simulink model "case2"  (R2024b)
settings: Solver=FixedStepAuto  StartTime=0  StopTime=1  FixedStep=1e-7  RelTol=1e-3
values from neighbouring files (symbols this model uses):
  SG_D_1_D = 0.01056    [IEEE9_case_parameters.m]    (also in case1_parameters.m; case2_parameters.m; case3_parameters.m; case4_parameters.m)
  SG_D_1_EnableSaturation = 0    [IEEE9_case_parameters.m]    (also in case1_parameters.m; case2_parameters.m; case3_parameters.m; case4_parameters.m)
  SG_D_1_f0 = 60    [IEEE9_case_parameters.m]    (also in case1_parameters.m; case2_parameters.m; case3_parameters.m; case4_parameters.m)
  SG_D_1_H = 7.5    [IEEE9_case_parameters.m]    (also in case1_parameters.m; case2_parameters.m; case3_parameters.m; case4_parameters.m)
  SG_D_1_K_A = 20    [IEEE9_case_parameters.m]    (also in case1_parameters.m; case2_parameters.m; case3_parameters.m; case4_parameters.m)
  SG_D_1_K_E = 1.000000e+1    (= 10)    [IEEE9_case_parameters.m]    (also in case1_parameters.m; case2_parameters.m; case3_parameters.m; case4_parameters.m)
  SG_D_1_K_F = 2.363    [IEEE9_case_parameters.m]    (also in case1_parameters.m; case2_parameters.m; case3_parameters.m; case4_parameters.m)
  SG_D_1_K_s = 0.5    [IEEE9_case_parameters.m]    (also in case1_parameters.m = 5; case2_parameters.m = 5; case3_parameters.m = 5; case4_parameters.m = 5)
  SG_D_1_R_a = 0.001088    [IEEE9_case_parameters.m]    (also in case1_parameters.m; case2_parameters.m; case3_parameters.m; case4_parameters.m)
  SG_D_1_S_A = 1    [IEEE9_case_parameters.m]    (also in case1_parameters.m; case2_parameters.m; case3_parameters.m; case4_parameters.m)
  SG_D_1_S_B = 0.103    [IEEE9_case_parameters.m]    (also in case1_parameters.m; case2_parameters.m; case3_parameters.m; case4_parameters.m)
  SG_D_1_S_N = 10.659857    [IEEE9_case_parameters.m]    (also in case1_parameters.m; case2_parameters.m; case3_parameters.m; case4_parameters.m)
  SG_D_1_SpeedPara = 200    [IEEE9_case_parameters.m]    (also in case1_parameters.m; case2_parameters.m; case3_parameters.m; case4_parameters.m)
  SG_D_1_T_0 = 0.720173    [IEEE9_case_parameters.m]    (also in case1_parameters.m = 0.755522; case2_parameters.m = 0.808931; case3_parameters.m = 0.869402; case4_parameters.m = 0.729316)
  SG_D_1_T_1 = 0.3    [IEEE9_case_parameters.m]    (also in case1_parameters.m; case2_parameters.m; case3_parameters.m; case4_parameters.m)
  SG_D_1_T_2 = 0.05    [IEEE9_case_parameters.m]    (also in case1_parameters.m; case2_parameters.m; case3_parameters.m; case4_parameters.m)
  SG_D_1_T_3 = 0.02    [IEEE9_case_parameters.m]    (also in case1_parameters.m; case2_parameters.m; case3_parameters.m; case4_parameters.m)
  SG_D_1_T_4 = 0.005    [IEEE9_case_parameters.m]    (also in case1_parameters.m; case2_parameters.m; case3_parameters.m; case4_parameters.m)
  SG_D_1_T_A = 0.02    [IEEE9_case_parameters.m]    (also in case1_parameters.m; case2_parameters.m; case3_parameters.m; case4_parameters.m)
  SG_D_1_T_dd = 8.000000e+0    (= 8)    [IEEE9_case_parameters.m]    (also in case1_parameters.m; case2_parameters.m; case3_parameters.m; case4_parameters.m)
  SG_D_1_T_ddd = 0.04    [IEEE9_case_parameters.m]    (also in case1_parameters.m; case2_parameters.m; case3_parameters.m; case4_parameters.m)
  SG_D_1_T_E = 0.314    [IEEE9_case_parameters.m]    (also in case1_parameters.m; case2_parameters.m; case3_parameters.m; case4_parameters.m)
  SG_D_1_T_F = 0.35    [IEEE9_case_parameters.m]    (also in case1_parameters.m; case2_parameters.m; case3_parameters.m; case4_parameters.m)
  SG_D_1_T_qd = 0.8    [IEEE9_case_parameters.m]    (also in case1_parameters.m; case2_parameters.m; case3_parameters.m; case4_parameters.m)
  SG_D_1_T_qdd = 0.02    [IEEE9_case_parameters.m]    (also in case1_parameters.m; case2_parameters.m; case3_parameters.m; case4_parameters.m)
  SG_D_1_T_speed = 0.1    [IEEE9_case_parameters.m]    (also in case1_parameters.m = 200; case2_parameters.m = 200; case3_parameters.m = 200; case4_parameters.m = 200)
  SG_D_1_T_w = 0.5    [IEEE9_case_parameters.m]    (also in case1_parameters.m; case2_parameters.m; case3_parameters.m; case4_parameters.m)
  SG_D_1_V_ref = 1.990276    [IEEE9_case_parameters.m]    (also in case1_parameters.m = 2.042296; case2_parameters.m = 2.051388; case3_parameters.m = 2.089584; case4_parameters.m = 2.01845)
  SG_D_1_w_ref = 376.991118    [IEEE9_case_parameters.m]    (also in case1_parameters.m; case2_parameters.m; case3_parameters.m; case4_parameters.m)
  SG_D_1_wb = 6.000000e+1    (= 60)    [IEEE9_case_parameters.m]    (also in case1_parameters.m; case2_parameters.m; case3_parameters.m; case4_parameters.m)
  SG_D_1_x_d = 1.9    [IEEE9_case_parameters.m]    (also in case1_parameters.m; case2_parameters.m; case3_parameters.m; case4_parameters.m)
  SG_D_1_x_dd = 0.302    [IEEE9_case_parameters.m]    (also in case1_parameters.m; case2_parameters.m; case3_parameters.m; case4_parameters.m)
  SG_D_1_x_ddd = 0.204    [IEEE9_case_parameters.m]    (also in case1_parameters.m; case2_parameters.m; case3_parameters.m; case4_parameters.m)
  SG_D_1_x_l = 0.05    [IEEE9_case_parameters.m]    (also in case1_parameters.m; case2_parameters.m; case3_parameters.m; case4_parameters.m)
  SG_D_1_x_q = 1.3    [IEEE9_case_parameters.m]    (also in case1_parameters.m; case2_parameters.m; case3_parameters.m; case4_parameters.m)
  SG_D_1_x_qd = 0.5    [IEEE9_case_parameters.m]    (also in case1_parameters.m; case2_parameters.m; case3_parameters.m; case4_parameters.m)
  SG_D_1_x_qdd = 0.3    [IEEE9_case_parameters.m]    (also in case1_parameters.m; case2_parameters.m; case3_parameters.m; case4_parameters.m)
  SG_D_2_D = 0.02    [IEEE9_case_parameters.m]    (also in case1_parameters.m; case2_parameters.m; case3_parameters.m; case4_parameters.m)
  SG_D_2_EnableSaturation = 0    [IEEE9_case_parameters.m]    (also in case1_parameters.m; case2_parameters.m; case3_parameters.m; case4_parameters.m)
  SG_D_2_f0 = 60    [IEEE9_case_parameters.m]    (also in case1_parameters.m; case2_parameters.m; case3_parameters.m; case4_parameters.m)
  SG_D_2_H = 8.000000e+0    (= 8)    [IEEE9_case_parameters.m]    (also in case1_parameters.m; case2_parameters.m; case3_parameters.m; case4_parameters.m)
  SG_D_2_K_A = 20    [IEEE9_case_parameters.m]    (also in case1_parameters.m; case2_parameters.m; case3_parameters.m; case4_parameters.m)
  SG_D_2_K_E = 1.000000e+1    (= 10)    [IEEE9_case_parameters.m]    (also in case1_parameters.m; case2_parameters.m; case3_parameters.m; case4_parameters.m)
  SG_D_2_K_F = 2.363    [IEEE9_case_parameters.m]    (also in case1_parameters.m; case2_parameters.m; case3_parameters.m; case4_parameters.m)
  SG_D_2_K_s = 0.5    [IEEE9_case_parameters.m]    (also in case1_parameters.m = 4; case2_parameters.m = 4; case3_parameters.m = 4; case4_parameters.m = 4)
  SG_D_2_R_a = 0.001088    [IEEE9_case_parameters.m]    (also in case1_parameters.m; case2_parameters.m; case3_parameters.m; case4_parameters.m)
  SG_D_2_S_A = 1    [IEEE9_case_parameters.m]    (also in case1_parameters.m; case2_parameters.m; case3_parameters.m; case4_parameters.m)
  SG_D_2_S_B = 0.103    [IEEE9_case_parameters.m]    (also in case1_parameters.m; case2_parameters.m; case3_parameters.m; case4_parameters.m)
  SG_D_2_S_N = 10.659857    [IEEE9_case_parameters.m]    (also in case1_parameters.m; case2_parameters.m; case3_parameters.m; case4_parameters.m)
  SG_D_2_SpeedPara = 200    [IEEE9_case_parameters.m]    (also in case1_parameters.m; case2_parameters.m; case3_parameters.m; case4_parameters.m)
  SG_D_2_T_0 = 1.632913    [IEEE9_case_parameters.m]    (also in case1_parameters.m = 1.632925; case2_parameters.m = 1.632915; case3_parameters.m = 1.632914; case4_parameters.m = 1.632927)
  SG_D_2_T_1 = 0.2    [IEEE9_case_parameters.m]    (also in case1_parameters.m; case2_parameters.m; case3_parameters.m; case4_parameters.m)
  SG_D_2_T_2 = 0.05    [IEEE9_case_parameters.m]    (also in case1_parameters.m; case2_parameters.m; case3_parameters.m; case4_parameters.m)
  SG_D_2_T_3 = 0.02    [IEEE9_case_parameters.m]    (also in case1_parameters.m; case2_parameters.m; case3_parameters.m; case4_parameters.m)
  SG_D_2_T_4 = 0.005    [IEEE9_case_parameters.m]    (also in case1_parameters.m; case2_parameters.m; case3_parameters.m; case4_parameters.m)
  SG_D_2_T_A = 0.02    [IEEE9_case_parameters.m]    (also in case1_parameters.m; case2_parameters.m; case3_parameters.m; case4_parameters.m)
  SG_D_2_T_dd = 7.9    [IEEE9_case_parameters.m]    (also in case1_parameters.m; case2_parameters.m; case3_parameters.m; case4_parameters.m)
  SG_D_2_T_ddd = 0.04    [IEEE9_case_parameters.m]    (also in case1_parameters.m; case2_parameters.m; case3_parameters.m; case4_parameters.m)
  SG_D_2_T_E = 0.314    [IEEE9_case_parameters.m]    (also in case1_parameters.m; case2_parameters.m; case3_parameters.m; case4_parameters.m)
  SG_D_2_T_F = 0.35    [IEEE9_case_parameters.m]    (also in case1_parameters.m; case2_parameters.m; case3_parameters.m; case4_parameters.m)
  SG_D_2_T_qd = 0.8    [IEEE9_case_parameters.m]    (also in case1_parameters.m; case2_parameters.m; case3_parameters.m; case4_parameters.m)
  SG_D_2_T_qdd = 0.015    [IEEE9_case_parameters.m]    (also in case1_parameters.m; case2_parameters.m; case3_parameters.m; case4_parameters.m)
  SG_D_2_T_speed = 0.1    [IEEE9_case_parameters.m]    (also in case1_parameters.m = 150; case2_parameters.m = 150; case3_parameters.m = 150; case4_parameters.m = 150)
  SG_D_2_T_w = 0.35    [IEEE9_case_parameters.m]    (also in case1_parameters.m; case2_parameters.m; case3_parameters.m; case4_parameters.m)
  SG_D_2_V_ref = 2.58547    [IEEE9_case_parameters.m]    (also in case1_parameters.m = 2.597896; case2_parameters.m = 2.587136; case3_parameters.m = 2.586042; case4_parameters.m = 2.599679)
  SG_D_2_w_ref = 376.991118    [IEEE9_case_parameters.m]    (also in case1_parameters.m; case2_parameters.m; case3_parameters.m; case4_parameters.m)
  SG_D_2_wb = 6.000000e+1    (= 60)    [IEEE9_case_parameters.m]    (also in case1_parameters.m; case2_parameters.m; case3_parameters.m; case4_parameters.m)
  SG_D_2_x_d = 1.8    [IEEE9_case_parameters.m]    (also in case1_parameters.m; case2_parameters.m; case3_parameters.m; case4_parameters.m)
  SG_D_2_x_dd = 0.302    [IEEE9_case_parameters.m]    (also in case1_parameters.m; case2_parameters.m; case3_parameters.m; case4_parameters.m)
  SG_D_2_x_ddd = 0.204    [IEEE9_case_parameters.m]    (also in case1_parameters.m; case2_parameters.m; case3_parameters.m; case4_parameters.m)
  SG_D_2_x_l = 0.05    [IEEE9_case_parameters.m]    (also in case1_parameters.m; case2_parameters.m; case3_parameters.m; case4_parameters.m)
  SG_D_2_x_q = 1.25    [IEEE9_case_parameters.m]    (also in case1_parameters.m; case2_parameters.m; case3_parameters.m; case4_parameters.m)
  SG_D_2_x_qd = 0.5    [IEEE9_case_parameters.m]    (also in case1_parameters.m; case2_parameters.m; case3_parameters.m; case4_parameters.m)
  SG_D_2_x_qdd = 0.3    [IEEE9_case_parameters.m]    (also in case1_parameters.m; case2_parameters.m; case3_parameters.m; case4_parameters.m)
  SG_D_3_D = 0.02    [IEEE9_case_parameters.m]    (also in case1_parameters.m; case2_parameters.m; case3_parameters.m; case4_parameters.m)
  SG_D_3_EnableSaturation = 0    [IEEE9_case_parameters.m]    (also in case1_parameters.m; case2_parameters.m; case3_parameters.m; case4_parameters.m)
  SG_D_3_f0 = 60    [IEEE9_case_parameters.m]    (also in case1_parameters.m; case2_parameters.m; case3_parameters.m; case4_parameters.m)
  SG_D_3_H = 7.7    [IEEE9_case_parameters.m]    (also in case1_parameters.m; case2_parameters.m; case3_parameters.m; case4_parameters.m)
  SG_D_3_K_A = 20    [IEEE9_case_parameters.m]    (also in case1_parameters.m; case2_parameters.m; case3_parameters.m; case4_parameters.m)
  SG_D_3_K_E = 1.000000e+1    (= 10)    [IEEE9_case_parameters.m]    (also in case1_parameters.m; case2_parameters.m; case3_parameters.m; case4_parameters.m)
  SG_D_3_K_F = 2.363    [IEEE9_case_parameters.m]    (also in case1_parameters.m; case2_parameters.m; case3_parameters.m; case4_parameters.m)
  SG_D_3_K_s = 0.2    [IEEE9_case_parameters.m]    (also in case1_parameters.m = 2; case2_parameters.m = 2; case3_parameters.m = 2; case4_parameters.m = 2)
  SG_D_3_R_a = 0.001088    [IEEE9_case_parameters.m]    (also in case1_parameters.m; case2_parameters.m; case3_parameters.m; case4_parameters.m)
  SG_D_3_S_A = 1    [IEEE9_case_parameters.m]    (also in case1_parameters.m; case2_parameters.m; case3_parameters.m; case4_parameters.m)
  SG_D_3_S_B = 0.103    [IEEE9_case_parameters.m]    (also in case1_parameters.m; case2_parameters.m; case3_parameters.m; case4_parameters.m)
  SG_D_3_S_N = 10.659857    [IEEE9_case_parameters.m]    (also in case1_parameters.m; case2_parameters.m; case3_parameters.m; case4_parameters.m)
  SG_D_3_SpeedPara = 200    [IEEE9_case_parameters.m]    (also in case1_parameters.m; case2_parameters.m; case3_parameters.m; case4_parameters.m)
  SG_D_3_T_0 = 0.850788    [IEEE9_case_parameters.m]    (also in case1_parameters.m = 0.850786; case2_parameters.m = 0.850787; case3_parameters.m; case4_parameters.m = 0.850786)
  SG_D_3_T_1 = 0.2    [IEEE9_case_parameters.m]    (also in case1_parameters.m; case2_parameters.m; case3_parameters.m; case4_parameters.m)
  SG_D_3_T_2 = 0.05    [IEEE9_case_parameters.m]    (also in case1_parameters.m; case2_parameters.m; case3_parameters.m; case4_parameters.m)
  SG_D_3_T_3 = 0.02    [IEEE9_case_parameters.m]    (also in case1_parameters.m; case2_parameters.m; case3_parameters.m; case4_parameters.m)
  SG_D_3_T_4 = 0.005    [IEEE9_case_parameters.m]    (also in case1_parameters.m; case2_parameters.m; case3_parameters.m; case4_parameters.m)
  SG_D_3_T_A = 0.02    [IEEE9_case_parameters.m]    (also in case1_parameters.m; case2_parameters.m; case3_parameters.m; case4_parameters.m)
  SG_D_3_T_dd = 8.1    [IEEE9_case_parameters.m]    (also in case1_parameters.m; case2_parameters.m; case3_parameters.m; case4_parameters.m)
  SG_D_3_T_ddd = 0.04    [IEEE9_case_parameters.m]    (also in case1_parameters.m; case2_parameters.m; case3_parameters.m; case4_parameters.m)
  SG_D_3_T_E = 0.314    [IEEE9_case_parameters.m]    (also in case1_parameters.m; case2_parameters.m; case3_parameters.m; case4_parameters.m)
  SG_D_3_T_F = 0.35    [IEEE9_case_parameters.m]    (also in case1_parameters.m; case2_parameters.m; case3_parameters.m; case4_parameters.m)
  SG_D_3_T_qd = 0.8    [IEEE9_case_parameters.m]    (also in case1_parameters.m; case2_parameters.m; case3_parameters.m; case4_parameters.m)
  SG_D_3_T_qdd = 0.015    [IEEE9_case_parameters.m]    (also in case1_parameters.m; case2_parameters.m; case3_parameters.m; case4_parameters.m)
  SG_D_3_T_speed = 0.1    [IEEE9_case_parameters.m]    (also in case1_parameters.m = 180; case2_parameters.m = 180; case3_parameters.m = 180; case4_parameters.m = 180)
  SG_D_3_T_w = 0.4    [IEEE9_case_parameters.m]    (also in case1_parameters.m; case2_parameters.m; case3_parameters.m; case4_parameters.m)
  SG_D_3_V_ref = 1.892727    [IEEE9_case_parameters.m]    (also in case1_parameters.m = 1.906439; case2_parameters.m = 1.895535; case3_parameters.m = 1.892105; case4_parameters.m = 1.906598)
  SG_D_3_w_ref = 376.991118    [IEEE9_case_parameters.m]    (also in case1_parameters.m; case2_parameters.m; case3_parameters.m; case4_parameters.m)
  SG_D_3_wb = 6.000000e+1    (= 60)    [IEEE9_case_parameters.m]    (also in case1_parameters.m; case2_parameters.m; case3_parameters.m; case4_parameters.m)
  SG_D_3_x_d = 1.85    [IEEE9_case_parameters.m]    (also in case1_parameters.m; case2_parameters.m; case3_parameters.m; case4_parameters.m)
  SG_D_3_x_dd = 0.302    [IEEE9_case_parameters.m]    (also in case1_parameters.m; case2_parameters.m; case3_parameters.m; case4_parameters.m)
  SG_D_3_x_ddd = 0.204    [IEEE9_case_parameters.m]    (also in case1_parameters.m; case2_parameters.m; case3_parameters.m; case4_parameters.m)
  SG_D_3_x_l = 0.05    [IEEE9_case_parameters.m]    (also in case1_parameters.m; case2_parameters.m; case3_parameters.m; case4_parameters.m)
  SG_D_3_x_q = 1.2    [IEEE9_case_parameters.m]    (also in case1_parameters.m; case2_parameters.m; case3_parameters.m; case4_parameters.m)
  SG_D_3_x_qd = 0.5    [IEEE9_case_parameters.m]    (also in case1_parameters.m; case2_parameters.m; case3_parameters.m; case4_parameters.m)
  SG_D_3_x_qdd = 0.3    [IEEE9_case_parameters.m]    (also in case1_parameters.m; case2_parameters.m; case3_parameters.m; case4_parameters.m)
(part 6 of 12)

== system case2/SG_D_1/d_psi_kq_SG_D_1_block ==
  note: d_psi_kq_SG_D_1 in case2
      | $-\frac{\psi _{\mathrm{gq},\mathrm{SG},D,1}+\psi _{\mathrm{kq},\mathrm{SG},D,1}+\frac{\left(x_{l}-x_{\mathrm{qd}}\right)\,\left(\psi _{q,\mathrm{SG},D,1}+\frac{\psi _{\mathrm{gq},\mathrm{SG},D,1}\,\left(x_{l}-x_{\mathrm{qdd}}\right)}{x_{l}-x_{\mathrm{qd}}}+\frac{\psi _{\mathrm{kq},\mathrm{SG},D,1}\,\left(x_{\mathrm{qd}}-x_{\mathrm{qdd}}\right)}{x_{l}-x_{\mathrm{qd}}}\right)}{x_{\mathrm{qdd}}}}{T_{\mathrm{qdd}}}$
      | Automatically generated on 2025-10-31 18:53:22 .
  State_psi_gq_SG_D_1_c4f58 : Inport
  State_psi_kq_SG_D_1_1e9b6 : Inport  Port=2
  State_psi_gq_SG_D_1_4c859 : Inport  Port=3
  State_psi_kq_SG_D_1_80b58 : Inport  Port=4
  State_psi_q_SG_D_1_7073d : Inport  Port=5
  Add_2bca2 : Sum
  Add_78ea9 : Sum
  Add_b1995 : Sum
  Add_cddc0 : Sum
  Add_d7741 : Sum
  Add_eedf9 : Sum
  Constant_-1_33263 : Constant  Value=-1
  Constant_-1_654fb : Constant  Value=-1
  Constant_-1_9578d : Constant  Value=-1
  Constant_-1_aaedf : Constant  Value=-1
  Constant_-1_e0c92 : Constant  Value=-1
  Constant_T_qdd_b3b24 : Constant  Value=T_qdd
  Constant_x_l_1c42c : Constant  Value=x_l
  Constant_x_l_1c86d : Constant  Value=x_l
  Constant_x_l_50126 : Constant  Value=x_l
  Constant_x_l_b4b36 : Constant  Value=x_l
  Constant_x_qd_3f0bc : Constant  Value=x_qd
  Constant_x_qd_b789d : Constant  Value=x_qd
  Constant_x_qd_bd3b2 : Constant  Value=x_qd
  Constant_x_qd_c3221 : Constant  Value=x_qd
  Constant_x_qdd_275e3 : Constant  Value=x_qdd
  Constant_x_qdd_64ab3 : Constant  Value=x_qdd
  Constant_x_qdd_e01a4 : Constant  Value=x_qdd
  Divide_020ec : Product  Inputs=*/
  Divide_3ab22 : Product  Inputs=*/
  Divide_65d3e : Product  Inputs=*/
  Divide_eedec : Product  Inputs=*/
  Product_466fa : Product
  Product_58b67 : Product
  Product_6d097 : Product
  Product_74f82 : Product
  Product_7c06e : Product
  Product_84edc : Product
  Product_a7cc4 : Product
  Product_df6af : Product
  Subtract_34d45 : Sum  Inputs=+-
  Subtract_946f3 : Sum  Inputs=+-
  Subtract_d6ec0 : Sum  Inputs=+-
  Blockout_d_psi_kq_SG_D_1_aa20d : Outport
  wires:
  Product_58b67/1 -> Add_b1995/1
  Constant_-1_aaedf/1 -> Product_58b67/1
  Constant_x_l_50126/1 -> Product_58b67/2
  Constant_x_qdd_64ab3/1 -> Add_b1995/2
  Constant_-1_9578d/1 -> Product_a7cc4/1
  Constant_x_qd_3f0bc/1 -> Subtract_d6ec0/1
  Constant_x_qd_bd3b2/1 -> Add_eedf9/2
  Constant_-1_33263/1 -> Product_6d097/1
  Constant_x_l_1c42c/1 -> Product_a7cc4/2
  Constant_x_qdd_e01a4/1 -> Subtract_d6ec0/2
  Constant_x_qd_c3221/1 -> Add_d7741/2
  Constant_x_l_1c86d/1 -> Product_6d097/2
  Subtract_34d45/1 -> Add_78ea9/1
  Product_7c06e/1 -> Subtract_34d45/1
  State_psi_gq_SG_D_1_4c859/1 -> Product_466fa/1
  Add_b1995/1 -> Product_466fa/2
  Product_6d097/1 -> Add_2bca2/1
  Constant_x_qd_b789d/1 -> Add_2bca2/2
  State_psi_kq_SG_D_1_80b58/1 -> Product_84edc/1
  Product_a7cc4/1 -> Add_d7741/1
  Subtract_d6ec0/1 -> Product_84edc/2
  Product_466fa/1 -> Divide_65d3e/1
  Add_2bca2/1 -> Divide_65d3e/2
  Product_84edc/1 -> Divide_3ab22/1
  Add_d7741/1 -> Divide_3ab22/2
  Constant_-1_e0c92/1 -> Product_df6af/1
  Constant_x_l_b4b36/1 -> Product_df6af/2
  Divide_65d3e/1 -> Subtract_946f3/1
  Divide_3ab22/1 -> Subtract_946f3/2
  Product_df6af/1 -> Add_eedf9/1
  Add_cddc0/1 -> Product_74f82/2
  Subtract_946f3/1 -> Add_cddc0/1
  State_psi_q_SG_D_1_7073d/1 -> Add_cddc0/2
  Constant_-1_654fb/1 -> Product_7c06e/1
  State_psi_gq_SG_D_1_c4f58/1 -> Product_7c06e/2
  Divide_eedec/1 -> Add_78ea9/2
  Product_74f82/1 -> Divide_eedec/1
  Add_eedf9/1 -> Product_74f82/1
  State_psi_kq_SG_D_1_1e9b6/1 -> Subtract_34d45/2
  Constant_x_qdd_275e3/1 -> Divide_eedec/2
  Add_78ea9/1 -> Divide_020ec/1
  Constant_T_qdd_b3b24/1 -> Divide_020ec/2
  Divide_020ec/1 -> Blockout_d_psi_kq_SG_D_1_aa20d/1

== system case2/SG_D_1/d_psi_q_SG_D_1_block ==
  note: d_psi_q_SG_D_1 in case2
      | $2\,\pi \,f_{0}\,\left(v_{d,\mathrm{SG},D,1}\,\cos\left(\theta _{\mathrm{SG},D,1}\right)+v_{q,\mathrm{SG},D,1}\,\sin\left(\theta _{\mathrm{SG},D,1}\right)-\frac{R_{a}\,\left(\psi _{q,\mathrm{SG},D,1}+\frac{\psi _{\mathrm{gq},\mathrm{SG},D,1}\,\left(x_{l}-x_{\mathrm{qdd}}\right)}{x_{l}-x_{\mathrm{qd}}}+\frac{\psi _{\mathrm{kq},\mathrm{SG},D,1}\,\left(x_{\mathrm{qd}}-x_{\mathrm{qdd}}\right)}{x_{l}-x_{\mathrm{qd}}}\right)}{x_{\mathrm{qdd}}}-\frac{\psi _{d,\mathrm{SG},D,1}\,w_{\mathrm{SG},D,1}}{2\,f_{0}\,\pi }\right)$
      | Automatically generated on 2025-10-31 18:53:04 .
  State_psi_gq_SG_D_1_6c5f8 : Inport
  State_psi_kq_SG_D_1_40857 : Inport  Port=2
  State_psi_q_SG_D_1_6bfdc : Inport  Port=3
  Input_v_d_SG_D_1_33d67 : Inport  Port=4
  State_theta_SG_D_1_0358b : Inport  Port=5
  Input_v_q_SG_D_1_717d9 : Inport  Port=6
  State_theta_SG_D_1_cb754 : Inport  Port=7
  State_psi_d_SG_D_1_19296 : Inport  Port=8
  State_w_SG_D_1_591a9 : Inport  Port=9
  Add_15bb5 : Sum
  Add_15e96 : Sum
  Add_61393 : Sum
  Add_771ae : Sum
  Add_93da0 : Sum
  Constant_-1_a4c86 : Constant  Value=-1
  Constant_-1_a677f : Constant  Value=-1
  Constant_-1_db15d : Constant  Value=-1
  Constant_-2.0_7ecc6 : Constant  Value=-2.0
  Constant_2.0_63966 : Constant  Value=2.0
  Constant_R_a_6f871 : Constant  Value=R_a
  Constant_f0_ea594 : Constant  Value=f0
  Constant_f0_f3201 : Constant  Value=f0
  Constant_pi_16e37 : Constant  Value=pi
  Constant_pi_6788c : Constant  Value=pi
  Constant_x_l_48838 : Constant  Value=x_l
  Constant_x_l_679d3 : Constant  Value=x_l
  Constant_x_l_cad5f : Constant  Value=x_l
  Constant_x_qd_91811 : Constant  Value=x_qd
  Constant_x_qd_abd0d : Constant  Value=x_qd
  Constant_x_qd_baaca : Constant  Value=x_qd
  Constant_x_qdd_847ba : Constant  Value=x_qdd
  Constant_x_qdd_d20cd : Constant  Value=x_qdd
  Constant_x_qdd_ffcdc : Constant  Value=x_qdd
  Divide_1fcbe : Product  Inputs=*/
  Divide_8395b : Product  Inputs=*/
  Divide_94cbe : Product  Inputs=*/
  Divide_c9c6d : Product  Inputs=*/
  MathFunc_cos_3d433 : Trigonometry  Operator=cos
  MathFunc_sin_f1ae6 : Trigonometry
  Product_0c8fc : Product
  Product_1b4b5 : Product
  Product_40790 : Product
  Product_68252 : Product
  Product_74441 : Product
  Product_89fe6 : Product
  Product_9bb0d : Product
  Product_a2ee6 : Product
  Product_a7a52 : Product
  Product_c3db8 : Product
  Product_c9e02 : Product
  Product_cc7e1 : Product
  Product_d0de8 : Product
  Product_e4c1d : Product
  Subtract_052e7 : Sum  Inputs=+-
  Subtract_2eb71 : Sum  Inputs=+-
  Subtract_908eb : Sum  Inputs=+-
  Subtract_ace0c : Sum  Inputs=+-
  Blockout_d_psi_q_SG_D_1_0c4c1 : Outport
  wires:
  Divide_94cbe/1 -> Subtract_ace0c/1
  Product_68252/1 -> Add_93da0/1
  Constant_x_l_679d3/1 -> Product_68252/2
  Constant_-1_a677f/1 -> Product_68252/1
  Constant_x_qdd_847ba/1 -> Add_93da0/2
  Constant_x_l_48838/1 -> Product_9bb0d/2
  Constant_-1_db15d/1 -> Product_9bb0d/1
  Constant_x_l_cad5f/1 -> Product_d0de8/2
  Constant_x_qdd_ffcdc/1 -> Subtract_908eb/2
  State_psi_kq_SG_D_1_40857/1 -> Product_74441/1
  Constant_-1_a4c86/1 -> Product_d0de8/1
  Constant_x_qd_abd0d/1 -> Subtract_908eb/1
  State_psi_gq_SG_D_1_6c5f8/1 -> Product_a2ee6/1
  Product_e4c1d/1 -> Blockout_d_psi_q_SG_D_1_0c4c1/1
  Subtract_ace0c/1 -> Add_61393/1
  Product_a2ee6/1 -> Divide_94cbe/1
  Add_93da0/1 -> Product_a2ee6/2
  Divide_1fcbe/1 -> Subtract_ace0c/2
  Product_9bb0d/1 -> Add_15e96/1
  Constant_x_qd_91811/1 -> Add_15e96/2
  Constant_-2.0_7ecc6/1 -> Product_0c8fc/1
  Product_74441/1 -> Divide_1fcbe/1
  Product_d0de8/1 -> Add_15bb5/1
  Subtract_908eb/1 -> Product_74441/2
  Constant_x_qd_baaca/1 -> Add_15bb5/2
  Add_15e96/1 -> Divide_94cbe/2
  Add_15bb5/1 -> Divide_1fcbe/2
  Constant_f0_f3201/1 -> Product_c3db8/2
  State_psi_q_SG_D_1_6bfdc/1 -> Add_61393/2
  Product_1b4b5/1 -> Product_89fe6/1
  Constant_R_a_6f871/1 -> Product_cc7e1/1
  Product_89fe6/1 -> Divide_8395b/2
  Product_cc7e1/1 -> Divide_c9c6d/1
  Add_61393/1 -> Product_cc7e1/2
  State_theta_SG_D_1_0358b/1 -> MathFunc_cos_3d433/1
  Input_v_d_SG_D_1_33d67/1 -> Product_c9e02/1
  Constant_x_qdd_d20cd/1 -> Divide_c9c6d/2
  MathFunc_cos_3d433/1 -> Product_c9e02/2
  State_theta_SG_D_1_cb754/1 -> MathFunc_sin_f1ae6/1
  Divide_c9c6d/1 -> Subtract_2eb71/1
  Constant_2.0_63966/1 -> Product_1b4b5/1
  State_w_SG_D_1_591a9/1 -> Product_40790/2
  Constant_pi_16e37/1 -> Product_1b4b5/2
  Subtract_052e7/1 -> Add_771ae/1
  Product_c9e02/1 -> Subtract_2eb71/2
  Divide_8395b/1 -> Add_771ae/2
  Input_v_q_SG_D_1_717d9/1 -> Product_a7a52/1
  MathFunc_sin_f1ae6/1 -> Product_a7a52/2
  Product_a7a52/1 -> Subtract_052e7/2
  State_psi_d_SG_D_1_19296/1 -> Product_40790/1
  Constant_f0_ea594/1 -> Product_89fe6/2
  Constant_pi_6788c/1 -> Product_0c8fc/2
  Subtract_2eb71/1 -> Subtract_052e7/1
  Product_40790/1 -> Divide_8395b/1
  Product_0c8fc/1 -> Product_c3db8/1
  Product_c3db8/1 -> Product_e4c1d/1
  Add_771ae/1 -> Product_e4c1d/2

== system case2/SG_D_1/d_theta_SG_D_1_block ==
  note: d_theta_SG_D_1 in case2
      | $w_{\mathrm{SG},D,1}-2\,\pi \,f_{0}$
      | Automatically generated on 2025-10-31 18:53:29 .
  State_w_SG_D_1_c2844 : Inport
  Add_5896a : Sum
  Constant_-2.0_4567a : Constant  Value=-2.0
  Constant_f0_1214b : Constant  Value=f0
  Constant_pi_355c3 : Constant  Value=pi
  Product_31175 : Product
  Product_91bed : Product
  Blockout_d_theta_SG_D_1_14305 : Outport
  wires:
  State_w_SG_D_1_c2844/1 -> Add_5896a/2
  Constant_-2.0_4567a/1 -> Product_91bed/1
  Constant_f0_1214b/1 -> Product_31175/2
  Constant_pi_355c3/1 -> Product_91bed/2
  Product_31175/1 -> Add_5896a/1
  Product_91bed/1 -> Product_31175/1
  Add_5896a/1 -> Blockout_d_theta_SG_D_1_14305/1

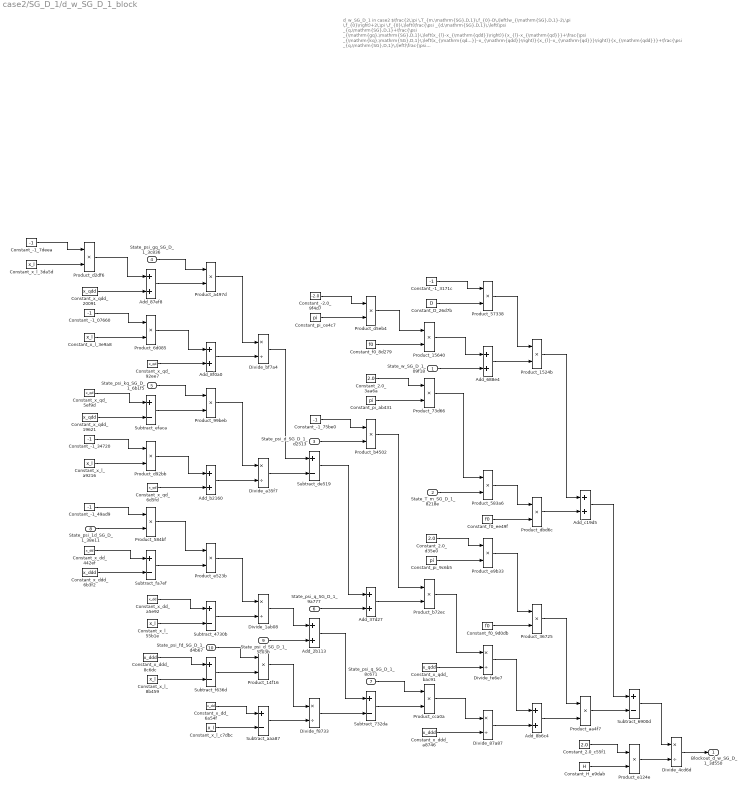
== system case2/SG_D_1/d_w_SG_D_1_block ==
  note: d_w_SG_D_1 in case2
      | $\frac{2\,\pi \,T_{m,\mathrm{SG},D,1}\,f_{0}-D\,\left(w_{\mathrm{SG},D,1}-2\,\pi \,f_{0}\right)+2\,\pi \,f_{0}\,\left(\frac{\psi _{d,\mathrm{SG},D,1}\,\left(\psi _{q,\mathrm{SG},D,1}+\frac{\psi _{\mathrm{gq},\mathrm{SG},D,1}\,\left(x_{l}-x_{\mathrm{qdd}}\right)}{x_{l}-x_{\mathrm{qd}}}+\frac{\psi _{\mathrm{kq},\mathrm{SG},D,1}\,\left(x_{\mathrm{qd}}-x_{\mathrm{qdd}}\right)}{x_{l}-x_{\mathrm{qd}}}\right)}{x_{\mathrm{qdd}}}+\frac{\psi _{q,\mathrm{SG},D,1}\,\left(\frac{\psi _{\mathrm{1d},\mathrm{SG},D,1}\,\left(x_{\mathrm{dd}}-x_{\mathrm{ddd}}\right)}{x_{\mathrm{dd}}-x_{l}}-\psi _{d,\mathrm{SG},D,1}+\frac{\psi _{\mathrm{fd},\mathrm{SG},D,1}\,\left(x_{\mathrm{ddd}}-x_{l}\right)}{x_{\mathrm{dd}}-x_{l}}\right)}{x_{\mathrm{ddd}}}\right)}{2\,H}$
      | Automatically generated on 2025-10-31 18:53:28 .
  State_w_SG_D_1_09f18 : Inport
  State_T_m_SG_D_1_8218e : Inport  Port=2
  State_psi_d_SG_D_1_d2513 : Inport  Port=3
  State_psi_gq_SG_D_1_3c836 : Inport  Port=4
  State_psi_kq_SG_D_1_6b1f5 : Inport  Port=5
  State_psi_q_SG_D_1_9a777 : Inport  Port=6
  State_psi_q_SG_D_1_8c671 : Inport  Port=7
  State_psi_1d_SG_D_1_38e11 : Inport  Port=8
  State_psi_d_SG_D_1_5c03b : Inport  Port=9
  State_psi_fd_SG_D_1_d4b67 : Inport  Port=10
  Add_2b113 : Sum
  Add_37d27 : Sum
  Add_688e4 : Sum
  Add_87ef8 : Sum
  Add_8b6c4 : Sum
  Add_8f0a0 : Sum
  Add_b2160 : Sum
  Add_c19d5 : Sum
  Constant_-1_07660 : Constant  Value=-1
  Constant_-1_3171c : Constant  Value=-1
  Constant_-1_34720 : Constant  Value=-1
  Constant_-1_49ad9 : Constant  Value=-1
  Constant_-1_75be0 : Constant  Value=-1
  Constant_-1_7deea : Constant  Value=-1
  Constant_-2.0_9f4d7 : Constant  Value=-2.0
  Constant_2.0_3aa6a : Constant  Value=2.0
  Constant_2.0_c55f1 : Constant  Value=2.0
  Constant_2.0_d35e0 : Constant  Value=2.0
  Constant_D_26d7b : Constant  Value=D
  Constant_H_e9dab : Constant  Value=H
  Constant_f0_8d279 : Constant  Value=f0
  Constant_f0_9d0db : Constant  Value=f0
  Constant_f0_ee49f : Constant  Value=f0
  Constant_pi_9c6b5 : Constant  Value=pi
  Constant_pi_ab431 : Constant  Value=pi
  Constant_pi_ce4c7 : Constant  Value=pi
  Constant_x_dd_442ef : Constant  Value=x_dd
  Constant_x_dd_6a54f : Constant  Value=x_dd
  Constant_x_dd_a5e92 : Constant  Value=x_dd
  Constant_x_ddd_6b3f2 : Constant  Value=x_ddd
  Constant_x_ddd_8c6dc : Constant  Value=x_ddd
  Constant_x_ddd_a8746 : Constant  Value=x_ddd
  Constant_x_l_3da5d : Constant  Value=x_l
  Constant_x_l_3e9a8 : Constant  Value=x_l
  Constant_x_l_55b1e : Constant  Value=x_l
  Constant_x_l_8b459 : Constant  Value=x_l
  Constant_x_l_a9216 : Constant  Value=x_l
  Constant_x_l_c7dbc : Constant  Value=x_l
  Constant_x_qd_5ef9d : Constant  Value=x_qd
  Constant_x_qd_6d5fd : Constant  Value=x_qd
  Constant_x_qd_92ee7 : Constant  Value=x_qd
  Constant_x_qdd_19621 : Constant  Value=x_qdd
  Constant_x_qdd_20091 : Constant  Value=x_qdd
  Constant_x_qdd_bac91 : Constant  Value=x_qdd
  Divide_1ab08 : Product  Inputs=*/
  Divide_4cd6d : Product  Inputs=*/
  Divide_87a87 : Product  Inputs=*/
  Divide_a35f7 : Product  Inputs=*/
  Divide_bf7a4 : Product  Inputs=*/
  Divide_f8733 : Product  Inputs=*/
  Divide_fe6e7 : Product  Inputs=*/
  Product_14f16 : Product
  Product_1524b : Product
  Product_15640 : Product
  Product_36725 : Product
  Product_57338 : Product
  Product_583a6 : Product
  Product_584bf : Product
  Product_6d085 : Product
  Product_73d66 : Product
  Product_99beb : Product
  Product_a497d : Product
  Product_aa4f7 : Product
  Product_b4502 : Product
  Product_b72ec : Product
  Product_cca0a : Product
  Product_d2df6 : Product
  Product_d5eb4 : Product
  Product_d92bb : Product
  Product_dbd6c : Product
  Product_e124e : Product
  Product_e523b : Product
  Product_e9b33 : Product
  Subtract_4730b : Sum  Inputs=+-
  Subtract_6900d : Sum  Inputs=+-
  Subtract_732da : Sum  Inputs=+-
  Subtract_aaa87 : Sum  Inputs=+-
  Subtract_de519 : Sum  Inputs=+-
  Subtract_efaca : Sum  Inputs=+-
  Subtract_f636d : Sum  Inputs=+-
  Subtract_fa7ef : Sum  Inputs=+-
  Blockout_d_w_SG_D_1_3d550 : Outport
  wires:
  Product_15640/1 -> Add_688e4/1
  Constant_-1_7deea/1 -> Product_d2df6/1
  Constant_pi_ab431/1 -> Product_73d66/2
  Constant_x_qdd_20091/1 -> Add_87ef8/2
  Constant_x_l_3da5d/1 -> Product_d2df6/2
  Product_d2df6/1 -> Add_87ef8/1
  Constant_x_qd_5ef9d/1 -> Subtract_efaca/1
  Constant_-1_07660/1 -> Product_6d085/1
  Product_d5eb4/1 -> Product_15640/1
  Constant_x_qdd_19621/1 -> Subtract_efaca/2
  State_psi_q_SG_D_1_8c671/1 -> Product_cca0a/1
  Constant_x_l_3e9a8/1 -> Product_6d085/2
  Constant_-1_34720/1 -> Product_d92bb/1
  Constant_x_l_a9216/1 -> Product_d92bb/2
  Constant_-1_49ad9/1 -> Product_584bf/1
  Product_6d085/1 -> Add_8f0a0/1
  State_psi_1d_SG_D_1_38e11/1 -> Product_584bf/2
  Constant_x_dd_442ef/1 -> Subtract_fa7ef/1
  Subtract_efaca/1 -> Product_99beb/2
  Constant_x_ddd_6b3f2/1 -> Subtract_fa7ef/2
  State_psi_gq_SG_D_1_3c836/1 -> Product_a497d/1
  Product_b4502/1 -> Product_b72ec/1
  Add_87ef8/1 -> Product_a497d/2
  Constant_x_qd_92ee7/1 -> Add_8f0a0/2
  State_psi_kq_SG_D_1_6b1f5/1 -> Product_99beb/1
  Constant_f0_8d279/1 -> Product_15640/2
  Product_d92bb/1 -> Add_b2160/1
  Constant_x_dd_a5e92/1 -> Subtract_4730b/1
  Constant_x_qd_6d5fd/1 -> Add_b2160/2
  Product_584bf/1 -> Product_e523b/1
  Subtract_fa7ef/1 -> Product_e523b/2
  Constant_x_l_55b1e/1 -> Subtract_4730b/2
  Constant_x_ddd_8c6dc/1 -> Subtract_f636d/1
  Constant_x_l_8b459/1 -> Subtract_f636d/2
  State_w_SG_D_1_09f18/1 -> Add_688e4/2
  Divide_fe6e7/1 -> Add_8b6c4/1
  Constant_-1_3171c/1 -> Product_57338/1
  Product_a497d/1 -> Divide_bf7a4/1
  Add_688e4/1 -> Product_1524b/2
  Divide_bf7a4/1 -> Subtract_de519/1
  Add_8f0a0/1 -> Divide_bf7a4/2
  Constant_pi_ce4c7/1 -> Product_d5eb4/2
  Product_99beb/1 -> Divide_a35f7/1
  Add_b2160/1 -> Divide_a35f7/2
  Product_e523b/1 -> Divide_1ab08/1
  Divide_1ab08/1 -> Add_2b113/1
  Subtract_4730b/1 -> Divide_1ab08/2
  State_psi_fd_SG_D_1_d4b67/1 -> Product_14f16/1
  Subtract_f636d/1 -> Product_14f16/2
  Constant_x_dd_6a54f/1 -> Subtract_aaa87/1
  Constant_x_l_c7dbc/1 -> Subtract_aaa87/2
  Divide_a35f7/1 -> Subtract_de519/2
  Constant_2.0_3aa6a/1 -> Product_73d66/1
  State_psi_d_SG_D_1_5c03b/1 -> Add_2b113/2
  Product_14f16/1 -> Divide_f8733/1
  Subtract_aaa87/1 -> Divide_f8733/2
  Constant_-2.0_9f4d7/1 -> Product_d5eb4/1
  Constant_-1_75be0/1 -> Product_b4502/1
  State_psi_d_SG_D_1_d2513/1 -> Product_b4502/2
  Subtract_de519/1 -> Add_37d27/1
  Subtract_732da/1 -> Product_cca0a/2
  State_psi_q_SG_D_1_9a777/1 -> Add_37d27/2
  Add_2b113/1 -> Subtract_732da/1
  Divide_f8733/1 -> Subtract_732da/2
  Add_37d27/1 -> Product_b72ec/2
  Constant_D_26d7b/1 -> Product_57338/2
  Product_73d66/1 -> Product_583a6/1
  State_T_m_SG_D_1_8218e/1 -> Product_583a6/2
  Constant_2.0_d35e0/1 -> Product_e9b33/1
  Constant_pi_9c6b5/1 -> Product_e9b33/2
  Product_b72ec/1 -> Divide_fe6e7/1
  Constant_x_qdd_bac91/1 -> Divide_fe6e7/2
  Product_cca0a/1 -> Divide_87a87/1
  Constant_x_ddd_a8746/1 -> Divide_87a87/2
  Product_57338/1 -> Product_1524b/1
  Product_583a6/1 -> Product_dbd6c/1
  Constant_f0_ee49f/1 -> Product_dbd6c/2
  Product_e9b33/1 -> Product_36725/1
  Constant_f0_9d0db/1 -> Product_36725/2
  Divide_87a87/1 -> Add_8b6c4/2
  Product_1524b/1 -> Add_c19d5/1
  Product_dbd6c/1 -> Add_c19d5/2
  Product_36725/1 -> Product_aa4f7/1
  Add_8b6c4/1 -> Product_aa4f7/2
  Add_c19d5/1 -> Subtract_6900d/1
  Product_aa4f7/1 -> Subtract_6900d/2
  Constant_2.0_c55f1/1 -> Product_e124e/1
  Constant_H_e9dab/1 -> Product_e124e/2
  Subtract_6900d/1 -> Divide_4cd6d/1
  Product_e124e/1 -> Divide_4cd6d/2
  Divide_4cd6d/1 -> Blockout_d_w_SG_D_1_3d550/1

== system case2/SG_D_1/i_d_SG_D_1_block ==
  note: i_d_SG_D_1 in case2
      | $\frac{\sin\left(\theta _{\mathrm{SG},D,1}\right)\,\left(\frac{\psi _{\mathrm{1d},\mathrm{SG},D,1}\,\left(x_{\mathrm{dd}}-x_{\mathrm{ddd}}\right)}{x_{\mathrm{dd}}-x_{l}}-\psi _{d,\mathrm{SG},D,1}+\frac{\psi _{\mathrm{fd},\mathrm{SG},D,1}\,\left(x_{\mathrm{ddd}}-x_{l}\right)}{x_{\mathrm{dd}}-x_{l}}\right)}{x_{\mathrm{ddd}}}-\frac{\cos\left(\theta _{\mathrm{SG},D,1}\right)\,\left(\psi _{q,\mathrm{SG},D,1}+\frac{\psi _{\mathrm{gq},\mathrm{SG},D,1}\,\left(x_{l}-x_{\mathrm{qdd}}\right)}{x_{l}-x_{\mathrm{qd}}}+\frac{\psi _{\mathrm{kq},\mathrm{SG},D,1}\,\left(x_{\mathrm{qd}}-x_{\mathrm{qdd}}\right)}{x_{l}-x_{\mathrm{qd}}}\right)}{x_{\mathrm{qdd}}}$
      | Automatically generated on 2025-10-31 18:53:51 .
  State_psi_gq_SG_D_1_57fbc : Inport
  State_psi_kq_SG_D_1_803a3 : Inport  Port=2
  State_psi_q_SG_D_1_70a4f : Inport  Port=3
  State_theta_SG_D_1_76dc5 : Inport  Port=4
  State_psi_1d_SG_D_1_4a4ce : Inport  Port=5
  State_psi_d_SG_D_1_bcca0 : Inport  Port=6
  State_psi_fd_SG_D_1_cd963 : Inport  Port=7
  State_theta_SG_D_1_6bfd9 : Inport  Port=8
  Add_7307d : Sum
  Add_9817a : Sum
  Add_ada8a : Sum
  Add_c9e55 : Sum
  Add_db9db : Sum
  Constant_-1_39fbe : Constant  Value=-1
  Constant_-1_425ea : Constant  Value=-1
  Constant_-1_67d53 : Constant  Value=-1
  Constant_-1_9033d : Constant  Value=-1
  Constant_-1_cc5da : Constant  Value=-1
  Constant_x_dd_4e5e2 : Constant  Value=x_dd
  Constant_x_dd_83ac0 : Constant  Value=x_dd
  Constant_x_dd_c4ccb : Constant  Value=x_dd
  Constant_x_ddd_35b96 : Constant  Value=x_ddd
  Constant_x_ddd_40f8d : Constant  Value=x_ddd
  Constant_x_ddd_e7ec2 : Constant  Value=x_ddd
  Constant_x_l_19407 : Constant  Value=x_l
  Constant_x_l_4bae3 : Constant  Value=x_l
  Constant_x_l_61b9b : Constant  Value=x_l
  Constant_x_l_8f2b5 : Constant  Value=x_l
  Constant_x_l_c1951 : Constant  Value=x_l
  Constant_x_l_ccb48 : Constant  Value=x_l
  Constant_x_qd_e63a9 : Constant  Value=x_qd
  Constant_x_qd_f13d0 : Constant  Value=x_qd
  Constant_x_qd_fa0b9 : Constant  Value=x_qd
  Constant_x_qdd_1fc6f : Constant  Value=x_qdd
  Constant_x_qdd_5aa75 : Constant  Value=x_qdd
  Constant_x_qdd_755ec : Constant  Value=x_qdd
  Divide_003ef : Product  Inputs=*/
  Divide_597a4 : Product  Inputs=*/
  Divide_6c0a4 : Product  Inputs=*/
  Divide_9375a : Product  Inputs=*/
  Divide_94be9 : Product  Inputs=*/
  Divide_cd470 : Product  Inputs=*/
  MathFunc_cos_7b7e3 : Trigonometry  Operator=cos
  MathFunc_sin_5b533 : Trigonometry
  Product_0f604 : Product
  Product_1447e : Product
  Product_2b389 : Product
  Product_37402 : Product
  Product_3a275 : Product
  Product_50d58 : Product
  Product_50f97 : Product
  Product_cff6b : Product
  Product_d3511 : Product
  Product_e8609 : Product
  Product_e92ef : Product
  Subtract_05412 : Sum  Inputs=+-
  Subtract_2650c : Sum  Inputs=+-
  Subtract_4c95e : Sum  Inputs=+-
  Subtract_5d98b : Sum  Inputs=+-
  Subtract_6f427 : Sum  Inputs=+-
  Subtract_a25a2 : Sum  Inputs=+-
  Subtract_ebf29 : Sum  Inputs=+-
  Subtract_ec599 : Sum  Inputs=+-
  Blockout_i_d_SG_D_1_7a741 : Outport
  wires:
  Constant_-1_425ea/1 -> Product_2b389/1
  Constant_x_l_19407/1 -> Product_2b389/2
  Constant_x_ddd_35b96/1 -> Subtract_ec599/2
  Product_2b389/1 -> Add_db9db/1
  Constant_x_qdd_755ec/1 -> Subtract_2650c/2
  Constant_x_l_4bae3/1 -> Product_37402/2
  Constant_x_qd_e63a9/1 -> Add_ada8a/2
  Constant_x_qdd_5aa75/1 -> Add_db9db/2
  Constant_x_qd_fa0b9/1 -> Subtract_2650c/1
  MathFunc_cos_7b7e3/1 -> Product_e92ef/2
  Constant_-1_39fbe/1 -> Product_37402/1
  Constant_-1_67d53/1 -> Product_e8609/1
  Subtract_a25a2/1 -> Blockout_i_d_SG_D_1_7a741/1
  Constant_x_l_ccb48/1 -> Product_e8609/2
  Divide_6c0a4/1 -> Subtract_05412/1
  State_psi_gq_SG_D_1_57fbc/1 -> Product_1447e/1
  Subtract_5d98b/1 -> Product_0f604/2
  Add_db9db/1 -> Product_1447e/2
  Divide_003ef/1 -> Add_7307d/1
  Product_37402/1 -> Add_9817a/1
  Constant_x_qd_f13d0/1 -> Add_9817a/2
  State_psi_kq_SG_D_1_803a3/1 -> Product_cff6b/1
  Add_7307d/1 -> Subtract_4c95e/1
  Add_9817a/1 -> Divide_6c0a4/2
  Subtract_2650c/1 -> Product_cff6b/2
  Product_e8609/1 -> Add_ada8a/1
  Constant_-1_9033d/1 -> Product_50f97/1
  State_psi_1d_SG_D_1_4a4ce/1 -> Product_50f97/2
  Constant_x_dd_c4ccb/1 -> Subtract_ec599/1
  Product_1447e/1 -> Divide_6c0a4/1
  Product_3a275/1 -> Divide_94be9/1
  Subtract_ec599/1 -> Product_d3511/2
  Product_cff6b/1 -> Divide_9375a/1
  Product_50f97/1 -> Product_d3511/1
  Add_ada8a/1 -> Divide_9375a/2
  Constant_x_dd_83ac0/1 -> Subtract_6f427/1
  Subtract_05412/1 -> Add_c9e55/1
  Constant_x_l_8f2b5/1 -> Subtract_6f427/2
  Constant_x_ddd_40f8d/1 -> Subtract_5d98b/1
  Constant_x_l_61b9b/1 -> Subtract_5d98b/2
  Divide_94be9/1 -> Subtract_a25a2/2
  Divide_9375a/1 -> Subtract_05412/2
  State_theta_SG_D_1_76dc5/1 -> MathFunc_cos_7b7e3/1
  Product_d3511/1 -> Divide_003ef/1
  Subtract_6f427/1 -> Divide_003ef/2
  State_theta_SG_D_1_6bfd9/1 -> MathFunc_sin_5b533/1
  State_psi_fd_SG_D_1_cd963/1 -> Product_0f604/1
  Constant_x_dd_4e5e2/1 -> Subtract_ebf29/1
  Constant_x_l_c1951/1 -> Subtract_ebf29/2
  State_psi_q_SG_D_1_70a4f/1 -> Add_c9e55/2
  State_psi_d_SG_D_1_bcca0/1 -> Add_7307d/2
  Constant_x_ddd_e7ec2/1 -> Divide_94be9/2
  MathFunc_sin_5b533/1 -> Product_3a275/2
  Product_0f604/1 -> Divide_597a4/1
  Constant_-1_cc5da/1 -> Product_50d58/1
  Subtract_ebf29/1 -> Divide_597a4/2
  Add_c9e55/1 -> Product_50d58/2
  Divide_597a4/1 -> Subtract_4c95e/2
  Product_50d58/1 -> Product_e92ef/1
  Subtract_4c95e/1 -> Product_3a275/1
  Constant_x_qdd_1fc6f/1 -> Divide_cd470/2
  Product_e92ef/1 -> Divide_cd470/1
  Divide_cd470/1 -> Subtract_a25a2/1

== system case2/SG_D_1/i_q_SG_D_1_block ==
  note: i_q_SG_D_1 in case2
      | $-\frac{\sin\left(\theta _{\mathrm{SG},D,1}\right)\,\left(\psi _{q,\mathrm{SG},D,1}+\frac{\psi _{\mathrm{gq},\mathrm{SG},D,1}\,\left(x_{l}-x_{\mathrm{qdd}}\right)}{x_{l}-x_{\mathrm{qd}}}+\frac{\psi _{\mathrm{kq},\mathrm{SG},D,1}\,\left(x_{\mathrm{qd}}-x_{\mathrm{qdd}}\right)}{x_{l}-x_{\mathrm{qd}}}\right)}{x_{\mathrm{qdd}}}-\frac{\cos\left(\theta _{\mathrm{SG},D,1}\right)\,\left(\frac{\psi _{\mathrm{1d},\mathrm{SG},D,1}\,\left(x_{\mathrm{dd}}-x_{\mathrm{ddd}}\right)}{x_{\mathrm{dd}}-x_{l}}-\psi _{d,\mathrm{SG},D,1}+\frac{\psi _{\mathrm{fd},\mathrm{SG},D,1}\,\left(x_{\mathrm{ddd}}-x_{l}\right)}{x_{\mathrm{dd}}-x_{l}}\right)}{x_{\mathrm{ddd}}}$
      | Automatically generated on 2025-10-31 18:53:55 .
  State_psi_gq_SG_D_1_8309b : Inport
  State_psi_kq_SG_D_1_9fa57 : Inport  Port=2
  State_psi_q_SG_D_1_72951 : Inport  Port=3
  State_theta_SG_D_1_5ff93 : Inport  Port=4
  State_psi_1d_SG_D_1_f4d32 : Inport  Port=5
  State_psi_d_SG_D_1_d1dd7 : Inport  Port=6
  State_psi_fd_SG_D_1_7071a : Inport  Port=7
  State_theta_SG_D_1_754c0 : Inport  Port=8
  Add_3009f : Sum
  Add_54f2e : Sum
  Add_7dba1 : Sum
  Add_7ec10 : Sum
  Add_bf609 : Sum
  Add_c1bbf : Sum
  Constant_-1_08132 : Constant  Value=-1
  Constant_-1_76745 : Constant  Value=-1
  Constant_-1_88916 : Constant  Value=-1
  Constant_-1_97a64 : Constant  Value=-1
  Constant_-1_c1df3 : Constant  Value=-1
  Constant_x_dd_a563b : Constant  Value=x_dd
  Constant_x_dd_b17bb : Constant  Value=x_dd
  Constant_x_dd_ccc61 : Constant  Value=x_dd
  Constant_x_ddd_6fbf0 : Constant  Value=x_ddd
  Constant_x_ddd_73170 : Constant  Value=x_ddd
  Constant_x_ddd_83015 : Constant  Value=x_ddd
  Constant_x_l_3564f : Constant  Value=x_l
  Constant_x_l_35b5e : Constant  Value=x_l
  Constant_x_l_5107a : Constant  Value=x_l
  Constant_x_l_56abb : Constant  Value=x_l
  Constant_x_l_a6a41 : Constant  Value=x_l
  Constant_x_l_bb42c : Constant  Value=x_l
  Constant_x_qd_0f9d7 : Constant  Value=x_qd
  Constant_x_qd_53a16 : Constant  Value=x_qd
  Constant_x_qd_6c068 : Constant  Value=x_qd
  Constant_x_qdd_08e39 : Constant  Value=x_qdd
  Constant_x_qdd_4f727 : Constant  Value=x_qdd
  Constant_x_qdd_93caa : Constant  Value=x_qdd
  Divide_3ef9e : Product  Inputs=*/
  Divide_4260f : Product  Inputs=*/
  Divide_4369d : Product  Inputs=*/
  Divide_47377 : Product  Inputs=*/
  Divide_e0a56 : Product  Inputs=*/
  Divide_fc4d5 : Product  Inputs=*/
  MathFunc_cos_4797b : Trigonometry  Operator=cos
  MathFunc_sin_20cb5 : Trigonometry
  Product_0488c : Product
  Product_0e625 : Product
  Product_14c03 : Product
  Product_1e28e : Product
  Product_30a47 : Product
  Product_58fad : Product
  Product_7478c : Product
  Product_7f0ea : Product
  Product_9d0e8 : Product
  Product_ca6fa : Product
  Product_ecd27 : Product
  Subtract_352f1 : Sum  Inputs=+-
  Subtract_44e57 : Sum  Inputs=+-
  Subtract_4bef5 : Sum  Inputs=+-
  Subtract_51f6f : Sum  Inputs=+-
  Subtract_58643 : Sum  Inputs=+-
  Subtract_5b2a0 : Sum  Inputs=+-
  Subtract_61c87 : Sum  Inputs=+-
  Blockout_i_q_SG_D_1_07e0d : Outport
  wires:
  State_theta_SG_D_1_754c0/1 -> MathFunc_cos_4797b/1
  State_psi_fd_SG_D_1_7071a/1 -> Product_30a47/1
  Constant_-1_c1df3/1 -> Product_14c03/1
  Constant_x_l_a6a41/1 -> Product_14c03/2
  Subtract_44e57/1 -> Product_30a47/2
  Constant_x_l_bb42c/1 -> Subtract_51f6f/2
  Product_14c03/1 -> Add_c1bbf/1
  Constant_x_qdd_08e39/1 -> Add_c1bbf/2
  Constant_x_qd_6c068/1 -> Subtract_58643/1
  Constant_x_qdd_93caa/1 -> Divide_e0a56/2
  MathFunc_sin_20cb5/1 -> Product_0e625/2
  Constant_-1_97a64/1 -> Product_7f0ea/1
  Constant_x_qdd_4f727/1 -> Subtract_58643/2
  Add_7dba1/1 -> Product_1e28e/2
  Product_ecd27/1 -> Divide_fc4d5/1
  Constant_x_l_35b5e/1 -> Product_7f0ea/2
  Constant_-1_76745/1 -> Product_9d0e8/1
  Constant_x_l_56abb/1 -> Product_9d0e8/2
  State_psi_gq_SG_D_1_8309b/1 -> Product_ecd27/1
  Add_c1bbf/1 -> Product_ecd27/2
  Divide_4260f/1 -> Add_54f2e/1
  Product_7f0ea/1 -> Add_7ec10/1
  Divide_e0a56/1 -> Add_3009f/1
  Constant_x_qd_53a16/1 -> Add_7ec10/2
  State_psi_kq_SG_D_1_9fa57/1 -> Product_ca6fa/1
  Add_54f2e/1 -> Subtract_352f1/1
  Subtract_58643/1 -> Product_ca6fa/2
  Divide_fc4d5/1 -> Subtract_4bef5/1
  Add_7ec10/1 -> Divide_fc4d5/2
  Product_9d0e8/1 -> Add_bf609/1
  Constant_x_qd_0f9d7/1 -> Add_bf609/2
  Constant_-1_08132/1 -> Product_7478c/1
  MathFunc_cos_4797b/1 -> Product_58fad/2
  Product_30a47/1 -> Divide_47377/1
  State_psi_1d_SG_D_1_f4d32/1 -> Product_7478c/2
  Constant_x_l_3564f/1 -> Subtract_5b2a0/2
  Constant_x_dd_b17bb/1 -> Subtract_61c87/1
  Divide_47377/1 -> Subtract_352f1/2
  Constant_x_ddd_83015/1 -> Subtract_61c87/2
  Product_58fad/1 -> Divide_3ef9e/1
  Product_ca6fa/1 -> Divide_4369d/1
  Product_7478c/1 -> Product_0488c/1
  Add_bf609/1 -> Divide_4369d/2
  Subtract_61c87/1 -> Product_0488c/2
  State_psi_d_SG_D_1_d1dd7/1 -> Add_54f2e/2
  Constant_x_dd_ccc61/1 -> Subtract_51f6f/1
  Constant_x_ddd_73170/1 -> Subtract_44e57/1
  Constant_x_l_5107a/1 -> Subtract_44e57/2
  Divide_3ef9e/1 -> Add_3009f/2
  Divide_4369d/1 -> Subtract_4bef5/2
  State_theta_SG_D_1_5ff93/1 -> MathFunc_sin_20cb5/1
  Product_0488c/1 -> Divide_4260f/1
  Subtract_51f6f/1 -> Divide_4260f/2
  Constant_x_dd_a563b/1 -> Subtract_5b2a0/1
  Subtract_4bef5/1 -> Add_7dba1/1
  State_psi_q_SG_D_1_72951/1 -> Add_7dba1/2
  Subtract_5b2a0/1 -> Divide_47377/2
  Subtract_352f1/1 -> Product_58fad/1
  Constant_-1_88916/1 -> Product_1e28e/1
  Product_1e28e/1 -> Product_0e625/1
  Product_0e625/1 -> Divide_e0a56/1
  Constant_x_ddd_6fbf0/1 -> Divide_3ef9e/2
  Add_3009f/1 -> Blockout_i_q_SG_D_1_07e0d/1

== system case2/SG_D_1/theta_SG_D_1_out_block ==
  note: theta_SG_D_1_out in case2
      | $\theta _{\mathrm{SG},D,1}$
      | Automatically generated on 2025-10-31 18:54:00 .
  State_theta_SG_D_1_087cb : Inport
  Blockout_theta_SG_D_1_out_5cdf6 : Outport
  wires:
  State_theta_SG_D_1_087cb/1 -> Blockout_theta_SG_D_1_out_5cdf6/1

== system case2/SG_D_1/w_SG_D_1_out_block ==
  note: w_SG_D_1_out in case2
      | $w_{\mathrm{SG},D,1}$
      | Automatically generated on 2025-10-31 18:54:00 .
  State_w_SG_D_1_30d0f : Inport
  Blockout_w_SG_D_1_out_1070a : Outport
  wires:
  State_w_SG_D_1_30d0f/1 -> Blockout_w_SG_D_1_out_1070a/1
